simulink model "AirbrakeFlightSim"  (R2024b)
settings: Solver=ode45  StartTime=0.0  StopTime=18  FixedStep=0.001  RelTol=1e-4  AbsTol=1e-6
model workspace (MAT data in the model file):
  test = 1
undefined symbols (not defined in the file or in its folder): accelerometer, atm, dspblkCoreblockFVToolHelper, gcbh, gyroscope, model_g_mps2, true_g_mps2, wn, zeta
libraries: simulink x14, simulink_extras x10, matrix_library x2, slpidlib x1
(part 1 of 2)
settings Model: Creator=colin  LastModifiedBy=colin
settings SolverCC: AutoScaleAbsTol=off
settings DebuggingCC: UnderSpecifiedDimensionMsg=warning

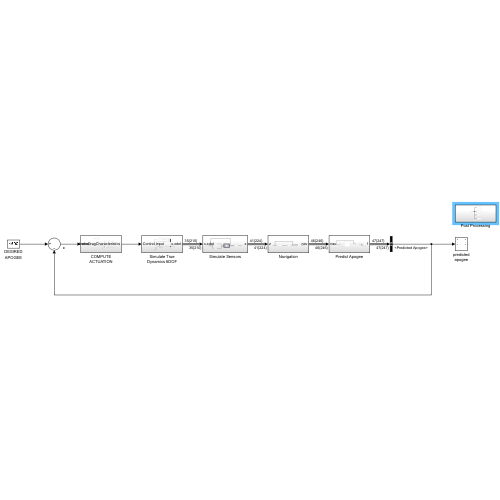
[thumbnail: Simulink's stored preview of the top-level diagram]
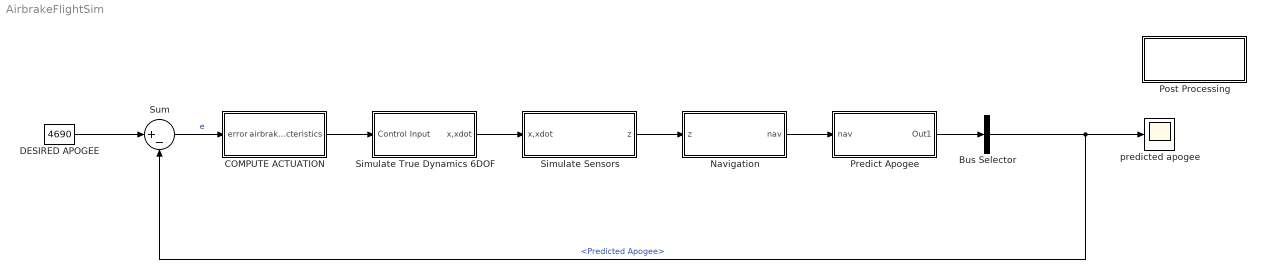
== system AirbrakeFlightSim ==
  Bus Selector : BusSelector  OutputSignals=Predicted Apogee
  COMPUTE ACTUATION : Subsystem
  DESIRED APOGEE : Constant  Value=4690
  Navigation : Subsystem
  Post Processing : Subsystem
  Predict Apogee : Subsystem
  Simulate Sensors : Subsystem
  Simulate True Dynamics 6DOF : Subsystem
  Sum : Sum  Inputs=|+-
  predicted apogee : Scope
  wires:
  DESIRED APOGEE/1 -> Sum/1
  Sum/1 -> COMPUTE ACTUATION/1(error)  "e"
  COMPUTE ACTUATION/1(airbrakeDragCharacteristics) -> Simulate True Dynamics 6DOF/1(Control Input)
  Simulate True Dynamics 6DOF/1(x,xdot) -> Simulate Sensors/1(x,xdot)
  Simulate Sensors/1(z) -> Navigation/1(z)
  Navigation/1(nav) -> Predict Apogee/1(nav)
  Bus Selector/1 -> predicted apogee/1, Sum/2  "<Predicted Apogee>"
  Predict Apogee/1(Out1) -> Bus Selector/1

== system AirbrakeFlightSim/COMPUTE ACTUATION ==
  error : Inport
  Add : Sum
  CONTROL SIGNAL : Scope
  CONTROLLER : slpidlib/PID Controller  Controller=PID  Form=Parallel  TimeDomain=Discrete-time  UseExternalTs=off  SampleTime=0.05  IntegratorMethod=Forward Euler  FilterMethod=Forward Euler  ControllerParametersSource=internal  P=10  I=1  UseKiTs=off  D=0  UseExternalDerivativeSource=off  N=0.01  UseFilter=on  TunerSelectOption=Frequency Response Based  InitialConditionSource=internal  InitialConditionForIntegrator=0  InitialConditionForFilter=0  DifferentiatorICPrevScaledInput=0  ExternalReset=none  TrackingMode=off  Kt=1  LimitOutput=off  SatLimitsSource=internal  UpperSaturationLimit=100  LowerSaturationLimit=0  LinearizeAsGain=on  AntiWindupMode=clamping  Kb=1  LimitIntegrator=off  UpperIntegratorSaturationLimit=inf  LowerIntegratorSaturationLimit=-inf  POutMin=[]  POutMax=[]  IOutMin=[]  IOutMax=[]  DOutMin=[]  DOutMax=[]  NOutMin=[]  NOutMax=[]  SumOutMin=[]  SumOutMax=[]  SaturationOutMin=[]  SaturationOutMax=[]  PParamMin=[]  PParamMax=[]  IParamMin=[]  IParamMax=[]  DParamMin=[]  DParamMax=[]  NParamMin=[]  NParamMax=[]  KbParamMin=[]  KbParamMax=[]  KtParamMin=[]  KtParamMax=[]  KbOutMin=[]  KbOutMax=[]  KtOutMin=[]  KtOutMax=[]  IntegratorOutMin=[]  IntegratorOutMax=[]  FilterOutMin=[]  FilterOutMax=[]  SumI1OutMin=[]  SumI1OutMax=[]  SumI2OutMin=[]  SumI2OutMax=[]  SumI3OutMin=[]  SumI3OutMax=[]  SumI4OutMin=[]  SumI4OutMax=[]  SumDOutMin=[]  SumDOutMax=[]  DifferentiatorOutMin=[]  DifferentiatorOutMax=[]  FilterDiffOutCoefMin=[]  FilterDiffOutCoefMax=[]  ReciprocalOutMin=[]  ReciprocalOutMax=[]  SumDenOutMin=[]  SumDenOutMax=[]  SumNumOutMin=[]  SumNumOutMax=[]  DivideOutMin=[]  DivideOutMax=[]  UdiffTsProdOutMin=[]  UdiffTsProdOutMax=[]  NTsProdOutMin=[]  NTsProdOutMax=[]  UintegralTsProdOutMin=[]  UintegralTsProdOutMax=[]  UngainTsProdOutMin=[]  UngainTsProdOutMax=[]  ClampingZeroOutDataTypeStr=Inherit: Inherit via back propagation  ClampingZeroOutMin=[]  ClampingZeroOutMax=[]  FilterDenConstantOutDataTypeStr=Inherit: Inherit via back propagation  FilterDenConstantOutMin=[]  FilterDenConstantOutMax=[]  PCopyOutDataTypeStr=Inherit: Inherit via back propagation  PCopyOutMin=[]  PCopyOutMax=[]  NCopyOutDataTypeStr=Inherit: Inherit via back propagation  NCopyOutMin=[]  NCopyOutMax=[]  IntegratorContinuousStateAttributes=''  IntegratorStateMustResolveToSignalObject=off  IntegratorRTWStateStorageClass=Auto  FilterContinuousStateAttributes=''  FilterStateMustResolveToSignalObject=off  FilterRTWStateStorageClass=Auto  ParallelPVariant=InternalParameters  IdealPVariant=Disabled  IVariant=InternalParameters  DVariant=InternalParameters  IntegratorVariant=Discrete  SatVariant=Disabled  AWVariant=Passthrough  PCopyVariant=Disabled  TRVariant=Disabled  FdbkBlocksVariant=Forward  IdealPFdbkVariant=Disabled  SatFdbkVariant=Disabled  DerivativeFilterVariant=ForwardEulerFilter  NVariant=InternalParameters  NCopyVariant=Disabled  FilterICVariant=InternalICsFilter  IntegratorICVariant=InternalICs  ExternalResetVariant=Disabled  TRSumVariant=Passthrough  SumFdbkVariant=Disabled  SumVariant=Sum_PID  TsampFilterVariant=InternalTs  TsampNgainVariant=Passthrough  TsampIntegralVariant=Disabled_SignalSpec  ExternalSaturationOutDataTypeStr=Inherit: Same as second input  DerivativeSourceVariant=ErrorSignal  PreIntVariant=InternalPreInt
  Cd*refArea2 : Constant  Value=0.00935787530743346
  DRAG : Scope
  ERROR SIGNAL : Scope
  GAIN-CONTROLLED SIGNAL : Scope
  Gain : Gain  Gain=-1
  Gain1 : Gain  Gain=-1e-4
  IDEAL DRAG : Scope
  Saturation1 : Saturate  UpperLimit=2*0.00935787530743346  LowerLimit=0.00935787530743346
  Switch1 : Switch  Criteria=u2 > Threshold  SaturateOnIntegerOverflow=off  InputSameDT=off
  airbrakeDragCharacteristics : Outport
  wires:
  CONTROLLER/1 -> Gain1/1, CONTROL SIGNAL/1
  Cd*refArea2/1 -> Add/2
  Gain1/1 -> GAIN-CONTROLLED SIGNAL/1, Add/1
  Add/1 -> Saturation1/1, IDEAL DRAG/1
  Saturation1/1 -> DRAG/1, airbrakeDragCharacteristics/1
  Gain/1 -> ERROR SIGNAL/1
  [motor_burnout] -> Switch1/2
  error/1 -> Switch1/1
  Switch1/1 -> CONTROLLER/1

== system AirbrakeFlightSim/Navigation ==
  z : Inport
  Compute Drag : Subsystem
  Dead Reckoning : Subsystem
  Reorganize : Subsystem
  nav : Outport
  wires:
  z/1 -> Dead Reckoning/1(z), Reorganize/1(z)
  Dead Reckoning/1(nav) -> Compute Drag/1(nav)
  Reorganize/1(Out1) -> nav/1
  Compute Drag/1(dragConstant) -> Reorganize/2(nav)

== system AirbrakeFlightSim/Post Processing ==
  Custom : Subsystem
  Navigation : Subsystem
  Navigation Error : Subsystem
  True Dynamics : Subsystem
  wires:
  [Master] -> True Dynamics/1(In1), Navigation/1(nav), Navigation Error/1(In1), Custom/1(In1)

== system AirbrakeFlightSim/Predict Apogee ==
  nav : Inport
  Bus Selector : BusSelector  OutputSignals=Navigation Data.Estimated Drag Constant,Navigation Data.NED.NED Velocity,Navigation Data.NED.NED Position
  PREDICT APOGEE : MATLAB Function  TreatAsAtomicUnit=on
  Reorganize : Subsystem
  Out1 : Outport
  tag scope: Master=global
  wires:
  Reorganize/1(Out1) -> Out1/1, [Master]
  PREDICT APOGEE/1(y) -> Reorganize/2(y)
  nav/1 -> Reorganize/1(nav), Bus Selector/1
  Bus Selector/3 -> PREDICT APOGEE/3(position)  "<NED Position>"
  Bus Selector/1 -> PREDICT APOGEE/1(dragConstant)  "<Estimated Drag Constant>"
  Bus Selector/2 -> PREDICT APOGEE/2(velocity)  "<NED Velocity>"

== system AirbrakeFlightSim/Simulate Sensors ==
  note: SELECT SENSOR MODE
  x,xdot : Inport
  Ideal Sensors : Subsystem
  Manual Switch : ManualSwitch
  Noisy Sensors : Subsystem
  Reorganize : Subsystem
  z : Outport
  wires:
  x,xdot/1 -> Noisy Sensors/1(x,xdot), Ideal Sensors/1(x,xdot), Reorganize/1(x,xdot)
  Ideal Sensors/1(meas) -> Manual Switch/2  "Ideal Measurements"
  Noisy Sensors/1(Measurements) -> Manual Switch/1
  Manual Switch/1 -> Reorganize/2(Measurements)  "Measurements"
  Reorganize/1(z) -> z/1

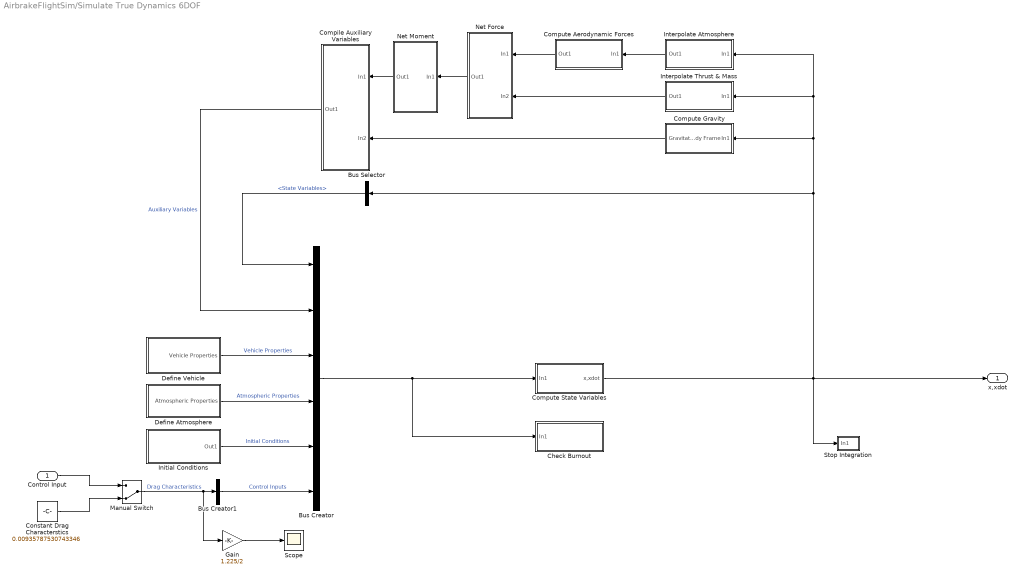
== system AirbrakeFlightSim/Simulate True Dynamics 6DOF ==
  Control Input : Inport
  Bus Creator : BusCreator  Inputs=State Variables,Auxiliary Variables,Vehicle Properties,Atmospheric Properties,Initial Conditions,Control Inputs
  Bus Creator1 : BusCreator  Inputs=Drag Characteristics
  Bus Selector : BusSelector  OutputSignals=State Variables
  Check Burnout : Subsystem
  Compile Auxiliary Variables : Subsystem
  Compute Aerodynamic Forces : Subsystem
  Compute Gravity : Subsystem
  Compute State Variables : Subsystem
  Constant Drag Characterstics : Constant  Value=0.00935787530743346
  Define Atmosphere : Subsystem
  Define Vehicle : Subsystem
  Gain : Gain  Gain=1.225/2
  Initial Conditions : Subsystem
  Interpolate Atmosphere : Subsystem
  Interpolate Thrust & Mass : Subsystem
  Manual Switch : ManualSwitch  CurrentSetting=0
  Net Force : Subsystem
  Net Moment : Subsystem
  Scope : Scope
  Stop Integration : Subsystem
  x,xdot : Outport
  wires:
  Compute Gravity/1(Gravitational Acceleration Vector in Body Frame) -> Compile Auxiliary Variables/2(In2)
  Define Vehicle/1(Vehicle Properties) -> Bus Creator/3  "Vehicle Properties"
  Initial Conditions/1(Out1) -> Bus Creator/5  "Initial Conditions"
  Bus Selector/1 -> Bus Creator/1  "<State Variables>"
  Compile Auxiliary Variables/1(Out1) -> Bus Creator/2  "Auxiliary Variables"
  Net Force/1(Out1) -> Net Moment/1(In1)
  Bus Creator/1 -> Compute State Variables/1(In1), Check Burnout/1(In1)
  Interpolate Thrust & Mass/1(Out1) -> Net Force/2(In2)
  Net Moment/1(Out1) -> Compile Auxiliary Variables/1(In1)
  Bus Creator1/1 -> Bus Creator/6  "Control Inputs"
  Manual Switch/1 -> Gain/1, Bus Creator1/1  "Drag Characteristics"
  Compute Aerodynamic Forces/1(Out1) -> Net Force/1(In1)
  Define Atmosphere/1(Atmospheric Properties) -> Bus Creator/4  "Atmospheric Properties"
  Interpolate Atmosphere/1(Out1) -> Compute Aerodynamic Forces/1(In1)
  Control Input/1 -> Manual Switch/1
  Constant Drag Characterstics/1 -> Manual Switch/2
  Compute State Variables/1(x,xdot) -> x,xdot/1, Stop Integration/1(In1), Bus Selector/1, Compute Gravity/1(In1), Interpolate Thrust & Mass/1(In1), Interpolate Atmosphere/1(In1)
  Gain/1 -> Scope/1

== system AirbrakeFlightSim/Navigation/Compute Drag ==
  nav : Inport
  Bus Selector : BusSelector  OutputSignals=NED.NED Acceleration,NED.NED Velocity
  MATLAB Function : MATLAB Function  TreatAsAtomicUnit=on
  Reorganize : Subsystem
  g NED1 : Constant  Value=[0 0 9.81]'
  dragConstant : Outport
  wires:
  nav/1 -> Bus Selector/1, Reorganize/1(nav)
  Reorganize/1(dragConstant) -> dragConstant/1
  MATLAB Function/1(drag_const) -> Reorganize/2(y)
  Bus Selector/1 -> MATLAB Function/1(a_ned_mps2)  "<NED Acceleration>"
  Bus Selector/2 -> MATLAB Function/2(v_ned_mps)  "<NED Velocity>"
  g NED1/1 -> MATLAB Function/3(gvec_ned)

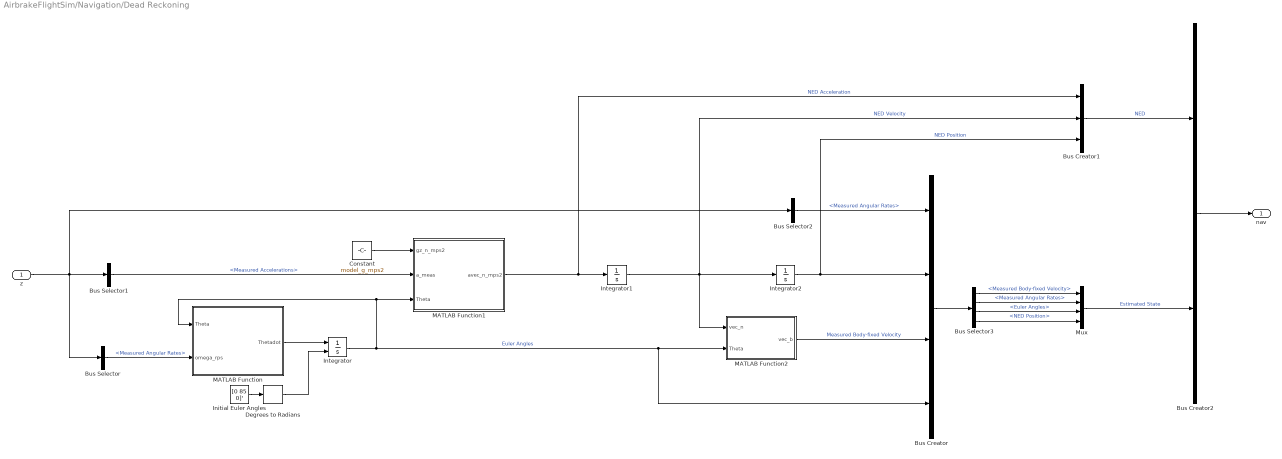
== system AirbrakeFlightSim/Navigation/Dead Reckoning ==
  z : Inport
  Bus Creator : BusCreator  Inputs=4
  Bus Creator1 : BusCreator  Inputs=3
  Bus Creator2 : BusCreator  Inputs=2
  Bus Selector : BusSelector  OutputSignals=Measurements.Measured Angular Rates
  Bus Selector1 : BusSelector  OutputSignals=Measurements.Measured Accelerations
  Bus Selector2 : BusSelector  OutputSignals=Measurements.Measured Angular Rates
  Bus Selector3 : BusSelector  OutputSignals=Measured Body-fixed Velocity,Measured Angular Rates,Euler Angles,NED Position
  Constant : Constant  Value=model_g_mps2
  Degrees to Radians : simulink_extras/Transformations/Degrees to Radians
  Initial Euler Angles : Constant  Value=[0 85 0]'
  Integrator : Integrator  InitialConditionSource=external
  Integrator1 : Integrator
  Integrator2 : Integrator
  MATLAB Function : MATLAB Function  TreatAsAtomicUnit=on
  MATLAB Function1 : MATLAB Function  TreatAsAtomicUnit=on
  MATLAB Function2 : MATLAB Function  TreatAsAtomicUnit=on
  Mux : Mux
  nav : Outport
  wires:
  Integrator2/1 -> Bus Creator/2, Bus Creator1/3  "NED Position"
  Integrator1/1 -> Bus Creator1/2, MATLAB Function2/1(vec_n), Integrator2/1  "NED Velocity"
  Integrator/1 -> Bus Creator/4, MATLAB Function2/2(Theta), MATLAB Function/1(Theta), MATLAB Function1/3(Theta)  "Euler Angles"
  Bus Selector3/4 -> Mux/4  "<NED Position>"
  MATLAB Function1/1(avec_n_mps2) -> Integrator1/1, Bus Creator1/1  "NED Acceleration"
  Degrees to Radians/1 -> Integrator/2
  z/1 -> Bus Selector2/1, Bus Selector1/1, Bus Selector/1
  Bus Creator/1 -> Bus Selector3/1
  Initial Euler Angles/1 -> Degrees to Radians/1
  Bus Selector2/1 -> Bus Creator/1  "<Measured Angular Rates>"
  MATLAB Function/1(Thetadot) -> Integrator/1
  Bus Selector/1 -> MATLAB Function/2(omega_rps)  "<Measured Angular Rates>"
  Bus Selector1/1 -> MATLAB Function1/2(a_meas)  "<Measured Accelerations>"
  Bus Selector3/3 -> Mux/3  "<Euler Angles>"
  MATLAB Function2/1(vec_b) -> Bus Creator/3  "Measured Body-fixed Velocity"
  Bus Selector3/2 -> Mux/2  "<Measured Angular Rates>"
  Bus Selector3/1 -> Mux/1  "<Measured Body-fixed Velocity>"
  Bus Creator1/1 -> Bus Creator2/1  "NED"
  Mux/1 -> Bus Creator2/2  "Estimated State"
  Bus Creator2/1 -> nav/1
  Constant/1 -> MATLAB Function1/1(gz_n_mps2)

== system AirbrakeFlightSim/Navigation/Reorganize ==
  z : Inport
  nav : Inport  Port=2
  Bus Creator : BusCreator  Inputs=8
  Bus Selector : BusSelector  OutputSignals=State Variables,State Derivatives,Vehicle Properties,Atmospheric Properties,Control Inputs,Auxiliary Variables,Measurements
  Out1 : Outport
  wires:
  z/1 -> Bus Selector/1
  Bus Selector/1 -> Bus Creator/1  "<State Variables>"
  Bus Selector/2 -> Bus Creator/2  "<State Derivatives>"
  Bus Selector/3 -> Bus Creator/3  "<Vehicle Properties>"
  Bus Selector/4 -> Bus Creator/4  "<Atmospheric Properties>"
  Bus Selector/5 -> Bus Creator/5  "<Control Inputs>"
  Bus Selector/6 -> Bus Creator/6  "<Auxiliary Variables>"
  Bus Selector/7 -> Bus Creator/7  "<Measurements>"
  nav/1 -> Bus Creator/8  "Navigation Data"
  Bus Creator/1 -> Out1/1

== system AirbrakeFlightSim/Post Processing/Custom ==
  In1 : Inport
  Bus Selector : BusSelector  OutputSignals=State Variables,State Derivatives,Auxiliary Variables.Simulation Time,Measurements.Measured GPS Position,Measurements.Measured GPS Velocity,Measurements.Measured Heading,Measurements.Measured Altitude,Measurements.Measured Angular Rates,Measurements.Measured Accelerations
  To Workspace : ToWorkspace  VariableName=x  SaveFormat=Timeseries  SampleTime=-1
  To Workspace1 : ToWorkspace  VariableName=xdot  SaveFormat=Timeseries  SampleTime=-1
  To Workspace2 : ToWorkspace  VariableName=t  SaveFormat=Timeseries  SampleTime=-1
  To Workspace3 : ToWorkspace  VariableName=gps_pos  SaveFormat=Timeseries  SampleTime=-1
  To Workspace4 : ToWorkspace  VariableName=gps_vel  SaveFormat=Timeseries  SampleTime=-1
  To Workspace5 : ToWorkspace  VariableName=mag_yaw  SaveFormat=Timeseries  SampleTime=-1
  To Workspace6 : ToWorkspace  VariableName=alti_pd  SaveFormat=Timeseries  SampleTime=-1
  To Workspace7 : ToWorkspace  VariableName=imu_pqr  SaveFormat=Timeseries  SampleTime=-1
  To Workspace8 : ToWorkspace  VariableName=imu_accel  SaveFormat=Timeseries  SampleTime=-1
  wires:
  In1/1 -> Bus Selector/1
  Bus Selector/1 -> To Workspace/1  "<State Variables>"
  Bus Selector/2 -> To Workspace1/1  "<State Derivatives>"
  Bus Selector/3 -> To Workspace2/1  "<Simulation Time>"
  Bus Selector/4 -> To Workspace3/1  "<Measured GPS Position>"
  Bus Selector/5 -> To Workspace4/1  "<Measured GPS Velocity>"
  Bus Selector/6 -> To Workspace5/1  "<Measured Heading>"
  Bus Selector/7 -> To Workspace6/1  "<Measured Altitude>"
  Bus Selector/8 -> To Workspace7/1  "<Measured Angular Rates>"
  Bus Selector/9 -> To Workspace8/1  "<Measured Accelerations>"

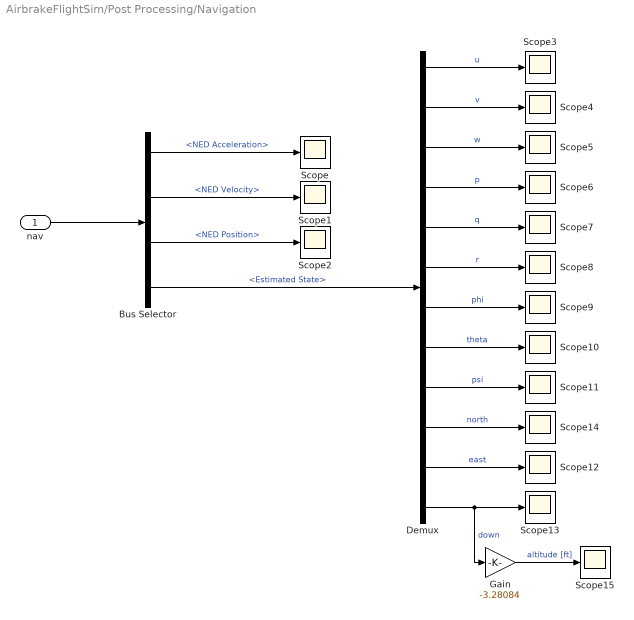
== system AirbrakeFlightSim/Post Processing/Navigation ==
  nav : Inport
  Bus Selector : BusSelector  OutputSignals=Navigation Data.NED.NED Acceleration,Navigation Data.NED.NED Velocity,Navigation Data.NED.NED Position,Navigation Data.Estimated State
  Demux : Demux  Outputs=12
  Gain : Gain  Gain=-3.28084
  Scope{,1..15} (16 alike) : Scope
  wires:
  Demux/8 -> Scope10/1  "theta"
  Demux/6 -> Scope8/1  "r"
  Demux/4 -> Scope6/1  "p"
  Demux/11 -> Scope12/1  "east"
  nav/1 -> Bus Selector/1
  Demux/5 -> Scope7/1  "q"
  Demux/3 -> Scope5/1  "w"
  Demux/2 -> Scope4/1  "v"
  Demux/10 -> Scope14/1  "north"
  Bus Selector/2 -> Scope1/1  "<NED Velocity>"
  Demux/7 -> Scope9/1  "phi"
  Demux/12 -> Gain/1, Scope13/1  "down"
  Demux/1 -> Scope3/1  "u"
  Bus Selector/4 -> Demux/1  "<Estimated State>"
  Bus Selector/1 -> Scope/1  "<NED Acceleration>"
  Demux/9 -> Scope11/1  "psi"
  Bus Selector/3 -> Scope2/1  "<NED Position>"
  Gain/1 -> Scope15/1  "altitude [ft]"

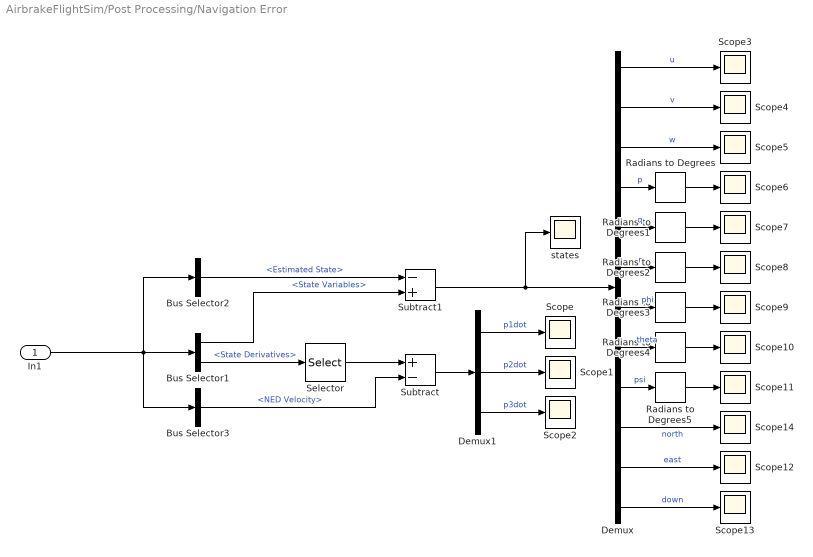
== system AirbrakeFlightSim/Post Processing/Navigation Error ==
  In1 : Inport
  Bus Selector1 : BusSelector  OutputSignals=State Variables,State Derivatives
  Bus Selector2 : BusSelector  OutputSignals=Navigation Data.Estimated State
  Bus Selector3 : BusSelector  OutputSignals=Navigation Data.NED.NED Velocity
  Demux : Demux  Outputs=12
  Demux1 : Demux  Outputs=3
  Radians to Degrees{,1..5} (6 alike) : simulink_extras/Transformations/Radians to Degrees
  Scope{,1..14} (15 alike) : Scope
  Selector : Selector  InputPortWidth=12  IndexOptions=Index vector (dialog)  Indices=[10 11 12]  OutputSizes=1
  Subtract : Sum  Inputs=+-
  Subtract1 : Sum  Inputs=-+
  states : Scope
  wires:
  In1/1 -> Bus Selector3/1, Bus Selector2/1, Bus Selector1/1
  Demux/4 -> Radians to Degrees/1  "p"
  Demux/12 -> Scope13/1  "down"
  Bus Selector1/2 -> Selector/1  "<State Derivatives>"
  Bus Selector2/1 -> Subtract1/1  "<Estimated State>"
  Subtract/1 -> Demux1/1
  Demux/5 -> Radians to Degrees1/1  "q"
  Demux/9 -> Radians to Degrees5/1  "psi"
  Bus Selector3/1 -> Subtract/2  "<NED Velocity>"
  Demux/3 -> Scope5/1  "w"
  Demux/1 -> Scope3/1  "u"
  Demux1/2 -> Scope1/1  "p2dot"
  Demux1/1 -> Scope/1  "p1dot"
  Demux1/3 -> Scope2/1  "p3dot"
  Demux/2 -> Scope4/1  "v"
  Demux/10 -> Scope14/1  "north"
  Subtract1/1 -> states/1, Demux/1
  Demux/6 -> Radians to Degrees2/1  "r"
  Bus Selector1/1 -> Subtract1/2  "<State Variables>"
  Demux/11 -> Scope12/1  "east"
  Selector/1 -> Subtract/1
  Demux/7 -> Radians to Degrees3/1  "phi"
  Demux/8 -> Radians to Degrees4/1  "theta"
  Radians to Degrees/1 -> Scope6/1
  Radians to Degrees1/1 -> Scope7/1
  Radians to Degrees2/1 -> Scope8/1
  Radians to Degrees3/1 -> Scope9/1
  Radians to Degrees4/1 -> Scope10/1
  Radians to Degrees5/1 -> Scope11/1

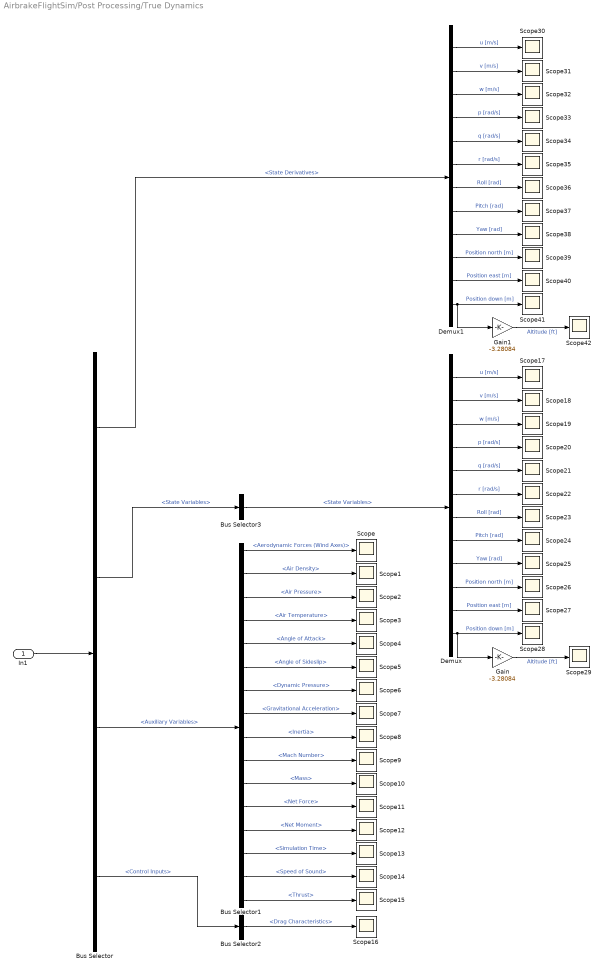
== system AirbrakeFlightSim/Post Processing/True Dynamics ==
  In1 : Inport
  Bus Selector : BusSelector  OutputSignals=State Derivatives,State Variables,Auxiliary Variables,Control Inputs
  Bus Selector1 : BusSelector  OutputSignals=Aerodynamic Forces (Wind Axes),Air Density,Air Pressure,Air Temperature,Angle of Attack,Angle of Sideslip,Dynamic Pressure,Gravitational Acceleration,Inertia,Mach Number,Mass,Net Force,Net Moment,Simulation Time,Speed of Sound,Thrust
  Bus Selector2 : BusSelector  OutputSignals=Drag Characteristics
  Bus Selector3 : BusSelector  OutputSignals=State Variables
  Demux : Demux  Outputs=12
  Demux1 : Demux  Outputs=12
  Gain : Gain  Gain=-3.28084
  Gain1 : Gain  Gain=-3.28084
  Scope{,1..42} (43 alike) : Scope
  wires:
  In1/1 -> Bus Selector/1
  Bus Selector/3 -> Bus Selector1/1  "<Auxiliary Variables>"
  Bus Selector/4 -> Bus Selector2/1  "<Control Inputs>"
  Bus Selector/2 -> Bus Selector3/1  "<State Variables>"
  Bus Selector1/1 -> Scope/1  "<Aerodynamic Forces (Wind Axes)>"
  Bus Selector1/2 -> Scope1/1  "<Air Density>"
  Bus Selector1/3 -> Scope2/1  "<Air Pressure>"
  Bus Selector3/1 -> Demux/1  "<State Variables>"
  Bus Selector2/1 -> Scope16/1  "<Drag Characteristics>"
  Bus Selector1/16 -> Scope15/1  "<Thrust>"
  Bus Selector1/15 -> Scope14/1  "<Speed of Sound>"
  Bus Selector1/14 -> Scope13/1  "<Simulation Time>"
  Bus Selector1/13 -> Scope12/1  "<Net Moment>"
  Bus Selector1/12 -> Scope11/1  "<Net Force>"
  Bus Selector1/11 -> Scope10/1  "<Mass>"
  Bus Selector1/10 -> Scope9/1  "<Mach Number>"
  Bus Selector1/9 -> Scope8/1  "<Inertia>"
  Bus Selector1/7 -> Scope6/1  "<Dynamic Pressure>"
  Bus Selector1/6 -> Scope5/1  "<Angle of Sideslip>"
  Bus Selector1/5 -> Scope4/1  "<Angle of Attack>"
  Bus Selector1/4 -> Scope3/1  "<Air Temperature>"
  Demux/1 -> Scope17/1  "u [m/s]"
  Demux/2 -> Scope18/1  "v [m/s]"
  Demux/3 -> Scope19/1  "w [m/s]"
  Demux/4 -> Scope20/1  "p [rad/s]"
  Demux/5 -> Scope21/1  "q [rad/s]"
  Demux/6 -> Scope22/1  "r [rad/s]"
  Demux/7 -> Scope23/1  "Roll [rad]"
  Demux/8 -> Scope24/1  "Pitch [rad]"
  Demux/9 -> Scope25/1  "Yaw [rad]"
  Demux/10 -> Scope26/1  "Position north [m]"
  Demux/11 -> Scope27/1  "Position east [m]"
  Demux/12 -> Scope28/1, Gain/1  "Position down [m]"
  Gain/1 -> Scope29/1  "Altitude [ft]"
  Bus Selector1/8 -> Scope7/1  "<Gravitational Acceleration>"
  Demux1/11 -> Scope40/1  "Position east [m]"
  Demux1/12 -> Scope41/1, Gain1/1  "Position down [m]"
  Demux1/2 -> Scope31/1  "v [m/s]"
  Demux1/9 -> Scope38/1  "Yaw [rad]"
  Demux1/7 -> Scope36/1  "Roll [rad]"
  Demux1/10 -> Scope39/1  "Position north [m]"
  Demux1/3 -> Scope32/1  "w [m/s]"
  Demux1/6 -> Scope35/1  "r [rad/s]"
  Demux1/5 -> Scope34/1  "q [rad/s]"
  Demux1/1 -> Scope30/1  "u [m/s]"
  Gain1/1 -> Scope42/1  "Altitude [ft]"
  Demux1/4 -> Scope33/1  "p [rad/s]"
  Demux1/8 -> Scope37/1  "Pitch [rad]"
  Bus Selector/1 -> Demux1/1  "<State Derivatives>"

== system AirbrakeFlightSim/Predict Apogee/Reorganize ==
  nav : Inport
  y : Inport  Port=2
  Bus Creator : BusCreator  Inputs=9
  Bus Selector : BusSelector  OutputSignals=State Variables,State Derivatives,Vehicle Properties,Atmospheric Properties,Control Inputs,Auxiliary Variables,Measurements,Navigation Data
  Out1 : Outport
  wires:
  nav/1 -> Bus Selector/1
  Bus Selector/1 -> Bus Creator/1  "<State Variables>"
  Bus Selector/2 -> Bus Creator/2  "<State Derivatives>"
  Bus Selector/3 -> Bus Creator/3  "<Vehicle Properties>"
  Bus Selector/4 -> Bus Creator/4  "<Atmospheric Properties>"
  Bus Selector/5 -> Bus Creator/5  "<Control Inputs>"
  Bus Selector/6 -> Bus Creator/6  "<Auxiliary Variables>"
  Bus Selector/8 -> Bus Creator/8  "<Navigation Data>"
  Bus Selector/7 -> Bus Creator/7  "<Measurements>"
  y/1 -> Bus Creator/9  "Predicted Apogee"
  Bus Creator/1 -> Out1/1

== system AirbrakeFlightSim/Simulate Sensors/Ideal Sensors ==
  x,xdot : Inport
  Altimeter : Subsystem
  Bus Creator : BusCreator  Inputs=6
  Bus Selector : BusSelector  OutputSignals=State Variables,State Derivatives
  CG to Accelerometer Position Vector [m] : Constant  Value=[0.2 0.05 -0.05]
  Constant : Constant  Value=true_g_mps2
  GPS : Subsystem
  MATLAB Function : MATLAB Function  TreatAsAtomicUnit=on
  Magnetometer : Subsystem
  Selector1 : Selector  InputPortWidth=12  IndexOptions=Index vector (dialog)  Indices=[4 5 6]  OutputSizes=1
  meas : Outport
  wires:
  x,xdot/1 -> GPS/1(x,xdot), Magnetometer/1(x,xdot), Altimeter/1(x,xdot), Bus Selector/1
  Bus Selector/1 -> Selector1/1, MATLAB Function/1(x)  "<State Variables>"
  Bus Selector/2 -> MATLAB Function/2(xdot)  "<State Derivatives>"
  CG to Accelerometer Position Vector [m]/1 -> MATLAB Function/3(r_b_sensor)
  Selector1/1 -> Bus Creator/5  "Measured Angular Rates"
  MATLAB Function/1(astar) -> Bus Creator/6  "Measured Accelerations"
  Bus Creator/1 -> meas/1
  Constant/1 -> MATLAB Function/4(gz_n_mps2)
  Altimeter/1(altitudehat) -> Bus Creator/4  "Measured Altitude"
  Magnetometer/1(headinghat) -> Bus Creator/3  "Measured Heading"
  GPS/2(vhat) -> Bus Creator/2  "Measured GPS Velocity"
  GPS/1(rhat) -> Bus Creator/1  "Measured GPS Position"

== system AirbrakeFlightSim/Simulate Sensors/Noisy Sensors ==
  note: Need to adjust these to be asynchronous
  x,xdot : Inport
  Accelerometer : Subsystem
  Altimeter : Subsystem
  Bus Creator : BusCreator  Inputs=6
  GPS : Subsystem
  Gyroscope : Subsystem
  Magnetometer : Subsystem
  Measurements : Outport
  wires:
  Altimeter/1(altitudehat) -> Bus Creator/4  "Measured Altitude"
  Gyroscope/1(omegahat) -> Bus Creator/5  "Measured Angular Rates"
  Accelerometer/1(ahat) -> Bus Creator/6  "Measured Accelerations"
  x,xdot/1 -> Accelerometer/1(x,xdot), Gyroscope/1(x,xdot), GPS/1(x,xdot), Magnetometer/1(x,xdot), Altimeter/1(x,xdot)
  Bus Creator/1 -> Measurements/1  "Measurements"
  Magnetometer/1(headinghat) -> Bus Creator/3  "Measured Heading"
  GPS/1(rhat) -> Bus Creator/1  "Measured GPS Position"
  GPS/2(vhat) -> Bus Creator/2  "Measured GPS Velocity"

== system AirbrakeFlightSim/Simulate Sensors/Reorganize ==
  x,xdot : Inport
  Measurements : Inport  Port=2
  Bus Creator : BusCreator  Inputs=7
  Bus Selector : BusSelector  OutputSignals=State Variables,State Derivatives,Vehicle Properties,Atmospheric Properties,Control Inputs,Auxiliary Variables
  z : Outport
  wires:
  x,xdot/1 -> Bus Selector/1
  Bus Selector/1 -> Bus Creator/1  "<State Variables>"
  Bus Selector/2 -> Bus Creator/2  "<State Derivatives>"
  Bus Selector/3 -> Bus Creator/3  "<Vehicle Properties>"
  Bus Selector/4 -> Bus Creator/4  "<Atmospheric Properties>"
  Bus Selector/5 -> Bus Creator/5  "<Control Inputs>"
  Bus Selector/6 -> Bus Creator/6  "<Auxiliary Variables>"
  Measurements/1 -> Bus Creator/7
  Bus Creator/1 -> z/1

== system AirbrakeFlightSim/Simulate True Dynamics 6DOF/Check Burnout ==
  In1 : Inport
  Add : Sum
  Add Constant : Bias  Bias=-0.1  SaturateOnIntegerOverflow=off
  Bus Selector : BusSelector  OutputSignals=Vehicle Properties.Motor Time Breakpoints,Auxiliary Variables.Simulation Time
  Gain : Gain  Gain=-1
  Selector : Selector  InputPortWidth=20  IndexOptions=Index vector (dialog)  Indices=[20]  OutputSizes=1
  tag scope: motor_burnout=global
  wires:
  Selector/1 -> Add/1
  Add/1 -> Add Constant/1  "Time Since Burnout"
  Bus Selector/1 -> Gain/1  "<Motor Time Breakpoints>"
  In1/1 -> Bus Selector/1
  Gain/1 -> Selector/1
  Bus Selector/2 -> Add/2  "<Simulation Time>"
  Add Constant/1 -> [motor_burnout]

== system AirbrakeFlightSim/Simulate True Dynamics 6DOF/Compile Auxiliary Variables ==
  In1 : Inport
  In2 : Inport  Port=2
  Bus Creator : BusCreator  Inputs=16
  Bus Selector : BusSelector  OutputSignals=Aerodynamic Forces (Wind Axes),Air Density,Air Pressure,Air Temperature,Angle of Attack,Angle of Sideslip,Dynamic Pressure,Inertia,Mach Number,Mass,Net Force,Net Moment,Simulation Time,Speed of Sound,Thrust
  Out1 : Outport
  wires:
  In1/1 -> Bus Selector/1
  In2/1 -> Bus Creator/8  "Gravitational Acceleration"
  Bus Selector/15 -> Bus Creator/16  "<Thrust>"
  Bus Selector/1 -> Bus Creator/1  "<Aerodynamic Forces (Wind Axes)>"
  Bus Selector/2 -> Bus Creator/2  "<Air Density>"
  Bus Selector/3 -> Bus Creator/3  "<Air Pressure>"
  Bus Selector/4 -> Bus Creator/4  "<Air Temperature>"
  Bus Selector/5 -> Bus Creator/5  "<Angle of Attack>"
  Bus Selector/6 -> Bus Creator/6  "<Angle of Sideslip>"
  Bus Selector/7 -> Bus Creator/7  "<Dynamic Pressure>"
  Bus Selector/8 -> Bus Creator/9  "<Inertia>"
  Bus Selector/9 -> Bus Creator/10  "<Mach Number>"
  Bus Selector/10 -> Bus Creator/11  "<Mass>"
  Bus Selector/11 -> Bus Creator/12  "<Net Force>"
  Bus Selector/12 -> Bus Creator/13  "<Net Moment>"
  Bus Selector/13 -> Bus Creator/14  "<Simulation Time>"
  Bus Selector/14 -> Bus Creator/15  "<Speed of Sound>"
  Bus Creator/1 -> Out1/1

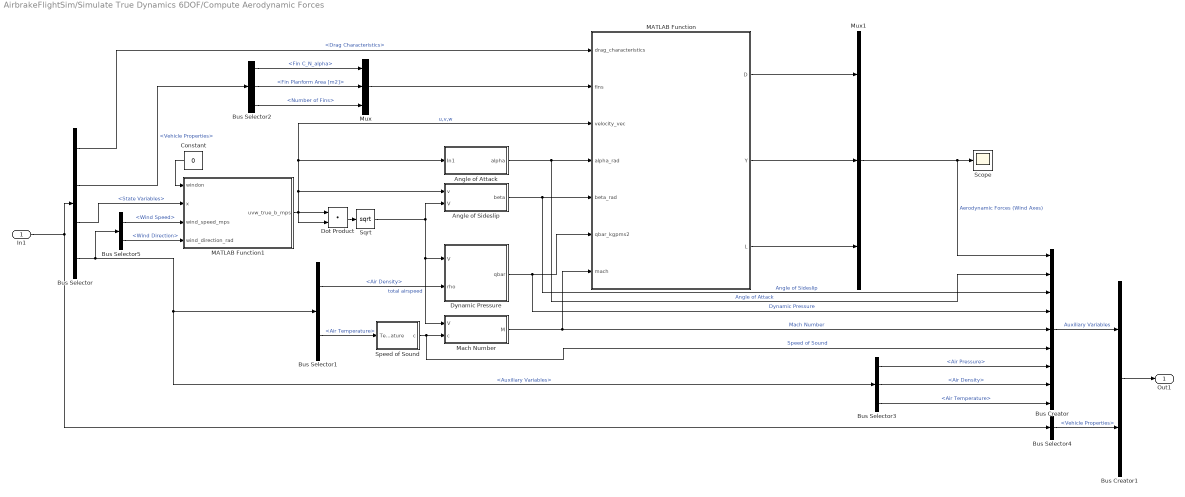
== system AirbrakeFlightSim/Simulate True Dynamics 6DOF/Compute Aerodynamic Forces ==
  In1 : Inport
  Angle of Attack : Subsystem
  Angle of Sideslip : Subsystem
  Bus Creator : BusCreator  Inputs=Aerodynamic Forces (Wind Axes),Angle of Attack,Angle of Sideslip,Dynamic Pressure,Mach Number,Speed of Sound,Air Pressure,Air Density,Air Temperature
  Bus Creator1 : BusCreator  Inputs=Auxiliary Variables,Vehicle Properties
  Bus Selector : BusSelector  OutputSignals=Control Inputs.Drag Characteristics,Vehicle Properties,State Variables,Auxiliary Variables
  Bus Selector1 : BusSelector  OutputSignals=Air Density,Air Temperature
  Bus Selector2 : BusSelector  OutputSignals=Fin C_N_alpha,Fin Planform Area [m2],Number of Fins
  Bus Selector3 : BusSelector  OutputSignals=Air Pressure,Air Density,Air Temperature
  Bus Selector4 : BusSelector  OutputSignals=Vehicle Properties
  Bus Selector5 : BusSelector  OutputSignals=Wind Speed,Wind Direction
  Constant : Constant  Value=0
  Dot Product : DotProduct  OutDataTypeStr=Inherit: Inherit via internal rule
  Dynamic Pressure : Subsystem
  MATLAB Function : MATLAB Function  TreatAsAtomicUnit=on
  MATLAB Function1 : MATLAB Function  TreatAsAtomicUnit=on
  Mach Number : Subsystem
  Mux : Mux  Inputs=3
  Mux1 : Mux  Inputs=3
  Scope : Scope
  Speed of Sound : Subsystem
  Sqrt : Sqrt
  Out1 : Outport
  wires:
  In1/1 -> Bus Selector4/1, Bus Selector/1
  MATLAB Function1/1(uvw_true_b_mps) -> Dot Product/2, MATLAB Function/3(velocity_vec), Angle of Attack/1(In1), Angle of Sideslip/1(v), Dot Product/1  "u,v,w"
  Sqrt/1 -> Dynamic Pressure/1(V), Mach Number/1(V), Angle of Sideslip/2(V)  "total airspeed"
  Dot Product/1 -> Sqrt/1
  Speed of Sound/1(c) -> Mach Number/2(c), Bus Creator/6  "Speed of Sound"
  Bus Selector/4 -> Bus Selector1/1, Bus Selector3/1, Bus Selector5/1  "<Auxiliary Variables>"
  Bus Selector1/1 -> Dynamic Pressure/2(rho)  "<Air Density>"
  Bus Selector1/2 -> Speed of Sound/1(Temperature)  "<Air Temperature>"
  Bus Selector/2 -> Bus Selector2/1  "<Vehicle Properties>"
  Angle of Attack/1(alpha) -> Bus Creator/2, MATLAB Function/4(alpha_rad)  "Angle of Attack"
  Angle of Sideslip/1(beta) -> Bus Creator/3, MATLAB Function/5(beta_rad)  "Angle of Sideslip"
  Dynamic Pressure/1(qbar) -> Bus Creator/4, MATLAB Function/6(qbar_kgpms2)  "Dynamic Pressure"
  Mach Number/1(M) -> Bus Creator/5, MATLAB Function/7(mach)  "Mach Number"
  Bus Selector2/3 -> Mux/3  "<Number of Fins>"
  Bus Selector2/2 -> Mux/2  "<Fin Planform Area [m2]>"
  Bus Selector2/1 -> Mux/1  "<Fin C_N_alpha>"
  Mux/1 -> MATLAB Function/2(fins)
  Bus Selector/1 -> MATLAB Function/1(drag_characteristics)  "<Drag Characteristics>"
  MATLAB Function/3(L) -> Mux1/3
  MATLAB Function/2(Y) -> Mux1/2
  MATLAB Function/1(D) -> Mux1/1
  Mux1/1 -> Scope/1, Bus Creator/1  "Aerodynamic Forces (Wind Axes)"
  Bus Selector3/1 -> Bus Creator/7  "<Air Pressure>"
  Bus Selector3/2 -> Bus Creator/8  "<Air Density>"
  Bus Selector3/3 -> Bus Creator/9  "<Air Temperature>"
  Bus Selector4/1 -> Bus Creator1/2  "<Vehicle Properties>"
  Bus Creator/1 -> Bus Creator1/1  "Auxiliary Variables"
  Bus Creator1/1 -> Out1/1
  Bus Selector/3 -> MATLAB Function1/2(x)  "<State Variables>"
  Bus Selector5/2 -> MATLAB Function1/4(wind_direction_rad)  "<Wind Direction>"
  Bus Selector5/1 -> MATLAB Function1/3(wind_speed_mps)  "<Wind Speed>"
  Constant/1 -> MATLAB Function1/1(windon)

== system AirbrakeFlightSim/Simulate True Dynamics 6DOF/Compute Gravity ==
  note: DCM_n2b_13
  note: NED to Body-Fixed
  note: Theta (Pitch) [rad]
  note: Phi (Roll) [rad]
  note: DCM_n2b_23
  note: DCM_n2b_33
  In1 : Inport
  Bus Selector : BusSelector  OutputSignals=State Variables
  Cos : Trigonometry  Operator=cos
  Cos1 : Trigonometry  Operator=cos
  Demux : Demux  Outputs=12
  Gain : Gain  Gain=-1
  Gain1 : Gain  Gain=true_g_mps2
  Gain2 : Gain  Gain=true_g_mps2
  Gain3 : Gain  Gain=true_g_mps2
  Mux : Mux  Inputs=3
  Product : Product
  Product1 : Product
  Sin : Trigonometry
  Sin1 : Trigonometry
  Gravitational Acceleration Vector in Body Frame : Outport
  wires:
  In1/1 -> Bus Selector/1
  Bus Selector/1 -> Demux/1  "<State Variables>"
  Demux/8 -> Cos1/1, Sin1/1
  Demux/7 -> Sin/1, Cos/1
  Sin1/1 -> Gain/1
  Sin/1 -> Product/1
  Cos1/1 -> Product1/1, Product/2
  Cos/1 -> Product1/2
  Gain/1 -> Gain1/1
  Product/1 -> Gain2/1
  Product1/1 -> Gain3/1
  Gain1/1 -> Mux/1
  Gain2/1 -> Mux/2
  Gain3/1 -> Mux/3
  Mux/1 -> Gravitational Acceleration Vector in Body Frame/1

== system AirbrakeFlightSim/Simulate True Dynamics 6DOF/Compute State Variables ==
  In1 : Inport
  Bus Creator1 : BusCreator  Inputs=6
  Bus Selector : BusSelector  OutputSignals=Vehicle Properties,Atmospheric Properties,Control Inputs,Auxiliary Variables
  Bus Selector1 : BusSelector  OutputSignals=State Variables,Auxiliary Variables.Net Force,Auxiliary Variables.Net Moment,Auxiliary Variables.Inertia,Auxiliary Variables.Mass,Auxiliary Variables.Gravitational Acceleration
  Bus Selector2 : BusSelector  OutputSignals=Initial Conditions.Initial State
  Integrator : Integrator  InitialConditionSource=external
  MATLAB Function : MATLAB Function  TreatAsAtomicUnit=on
  x,xdot : Outport
  wires:
  In1/1 -> Bus Selector/1, Bus Selector2/1, Bus Selector1/1
  Bus Creator1/1 -> x,xdot/1
  Bus Selector/1 -> Bus Creator1/3  "<Vehicle Properties>"
  Bus Selector/2 -> Bus Creator1/4  "<Atmospheric Properties>"
  Bus Selector/3 -> Bus Creator1/5  "<Control Inputs>"
  Bus Selector1/6 -> MATLAB Function/6(gvec_b_mps2)  "<Gravitational Acceleration>"
  Bus Selector1/5 -> MATLAB Function/5(m_kg)  "<Mass>"
  Bus Selector1/4 -> MATLAB Function/4(J_tensor_b_kgm2)  "<Inertia>"
  Bus Selector1/3 -> MATLAB Function/3(Mvec_b_N)  "<Net Moment>"
  Bus Selector1/2 -> MATLAB Function/2(Fvec_b_N)  "<Net Force>"
  Bus Selector1/1 -> MATLAB Function/1(x)  "<State Variables>"
  MATLAB Function/1(xdot) -> Integrator/1, Bus Creator1/2  "State Derivatives"
  Integrator/1 -> Bus Creator1/1  "State Variables"
  Bus Selector2/1 -> Integrator/2  "<Initial State>"
  Bus Selector/4 -> Bus Creator1/6  "<Auxiliary Variables>"

== system AirbrakeFlightSim/Simulate True Dynamics 6DOF/Define Atmosphere ==
  Bus Creator : BusCreator  Inputs=6
  Constant : Constant  Value=atm.elevation
  Constant1 : Constant  Value=atm.heights
  Constant2 : Constant  Value=atm.pressures
  Constant3 : Constant  Value=atm.temperatures
  Constant4 : Constant  Value=atm.wind_directions
  Constant5 : Constant  Value=atm.wind_speeds
  Atmospheric Properties : Outport
  wires:
  Bus Creator/1 -> Atmospheric Properties/1
  Constant/1 -> Bus Creator/1  "Local Elevation"
  Constant1/1 -> Bus Creator/2  "Height Breakpoints"
  Constant2/1 -> Bus Creator/3  "Pressure Breakpoints"
  Constant3/1 -> Bus Creator/4  "Temperature Breakpoints"
  Constant4/1 -> Bus Creator/5  "Wind Direction Breakpoints"
  Constant5/1 -> Bus Creator/6  "Wind Speed Breakpoints"

== system AirbrakeFlightSim/Simulate True Dynamics 6DOF/Define Vehicle ==
  note: Motor Properties
  note: Fins
  note: Geometric Properties
  note: Mass Properties
  note: Vehicle Mass in unloaded
      | configuration
  Bus Creator : BusCreator  Inputs=Vehicle Mass [kg],Vehicle Inertia [kg-m2],CG2CP Vector [m],Cross Sectional Area [m2],Number of Fins,Fin C_N_alpha,Fin Planform Area [m2],Motor Thrust Breakpoints,Motor Mass Breakpoints,Motor Time Breakpoints
  CG2CP Vector [m] : Constant  Value=[-0.5 0 0]
  Cross Sectional Area [m2] : Constant  Value=0.0154675624916256
  Fin C_N_alpha : Constant  Value=2.316
  Fin Planform Area [m2] : Constant  Value=0.02049724
  Motor Mass Breakpoints : Constant  Value=|
      | [   3.8555e+00
      |    3.8464e+00
      |    3.8325e+00
      |    3.8156e+00
      |    3.7411e+00
      |    3.5246e+00
      |    3.2573e+00
      |    2.9946e+00
      |    2.6223e+00
      |    2.3868e+00
      |    2.1980e+00
      |    2.1014e+00
      |    2.0699e+00
      |    2.0616e+00
      |    2.0533e+00
      |    2.0440e+00
      |    2.0356e+00
      |    2.0334e+00
      |    2.0321e+00
      |    2.0321e+00]
  Motor Thrust Breakpoints : Constant  Value=|
      | [   4.8137e+01
      |    2.1073e+03
      |    2.2892e+03
      |    2.1501e+03
      |    2.1020e+03
      |    2.1501e+03
      |    2.1555e+03
      |    2.1180e+03
      |    2.0004e+03
      |    1.8987e+03
      |    1.8399e+03
      |    1.8185e+03
      |    1.6527e+03
      |    1.3746e+03
      |    9.3600e+02
      |    5.3486e+02
      |    2.4069e+02
      |    1.1232e+02
      |    5.3490e+00
      |             0]
  Motor Time Breakpoints : Constant  Value=|
      | [   2.0000e-02
      |    4.0000e-02
      |    5.5000e-02
      |    7.3000e-02
      |    1.5600e-01
      |    3.9700e-01
      |    6.9100e-01
      |    9.8200e-01
      |    1.4100e+00
      |    1.6960e+00
      |    1.9350e+00
      |    2.0600e+00
      |    2.1030e+00
      |    2.1160e+00
      |    2.1330e+00
      |    2.1630e+00
      |    2.2140e+00
      |    2.2440e+00
      |    2.2960e+00
      |    2.3090e+00]
  Number of Fins : Constant  Value=3
  Vehicle Inertia [kg-m2] : Constant  Value=[9.2e-2 0 0; 0 19 0; 0 0 19]
  Vehicle Mass [kg] : Constant  Value=16.66100115
  Vehicle Properties : Outport
  wires:
  Vehicle Mass [kg]/1 -> Bus Creator/1  "Vehicle Mass [kg]"
  Vehicle Inertia [kg-m2]/1 -> Bus Creator/2  "Vehicle Inertia [kg-m2]"
  CG2CP Vector [m]/1 -> Bus Creator/3  "CG2CP Vector [m]"
  Cross Sectional Area [m2]/1 -> Bus Creator/4  "Cross Sectional Area [m2]"
  Number of Fins/1 -> Bus Creator/5  "Number of Fins"
  Fin C_N_alpha/1 -> Bus Creator/6  "Fin C_N_alpha"
  Fin Planform Area [m2]/1 -> Bus Creator/7  "Fin Planform Area [m2]"
  Motor Thrust Breakpoints/1 -> Bus Creator/8  "Motor Thrust Breakpoints"
  Motor Mass Breakpoints/1 -> Bus Creator/9  "Motor Mass Breakpoints"
  Motor Time Breakpoints/1 -> Bus Creator/10  "Motor Time Breakpoints"
  Bus Creator/1 -> Vehicle Properties/1  "Vehicle Properties"

== system AirbrakeFlightSim/Simulate True Dynamics 6DOF/Initial Conditions ==
  note: Initial State Vector
  note: Launch Rail Conditions
  Azimuth [deg] : Constant  Value=0
  Bus Creator : BusCreator  Inputs=Initial State
  Degrees to Radians : simulink_extras/Transformations/Degrees to Radians
  Degrees to Radians1 : simulink_extras/Transformations/Degrees to Radians
  Elevation [deg] : Constant  Value=85
  Mux : Mux  Inputs=12
  p0 : Constant  Value=0
  p_down_0 : Constant  Value=0
  p_east_0 : Constant  Value=0
  p_north_0 : Constant  Value=0
  phi0 : Constant  Value=0
  q0 : Constant  Value=0
  r0 : Constant  Value=0
  u0 : Constant  Value=0
  v0 : Constant  Value=0
  w0 : Constant  Value=0
  Out1 : Outport
  wires:
  u0/1 -> Mux/1
  v0/1 -> Mux/2
  w0/1 -> Mux/3
  p0/1 -> Mux/4
  q0/1 -> Mux/5
  r0/1 -> Mux/6
  Azimuth [deg]/1 -> Degrees to Radians/1
  p_north_0/1 -> Mux/10
  p_east_0/1 -> Mux/11
  p_down_0/1 -> Mux/12
  Elevation [deg]/1 -> Degrees to Radians1/1
  phi0/1 -> Mux/7
  Bus Creator/1 -> Out1/1
  Mux/1 -> Bus Creator/1  "Initial State"
  Degrees to Radians/1 -> Mux/9  "psi0"
  Degrees to Radians1/1 -> Mux/8  "theta0"

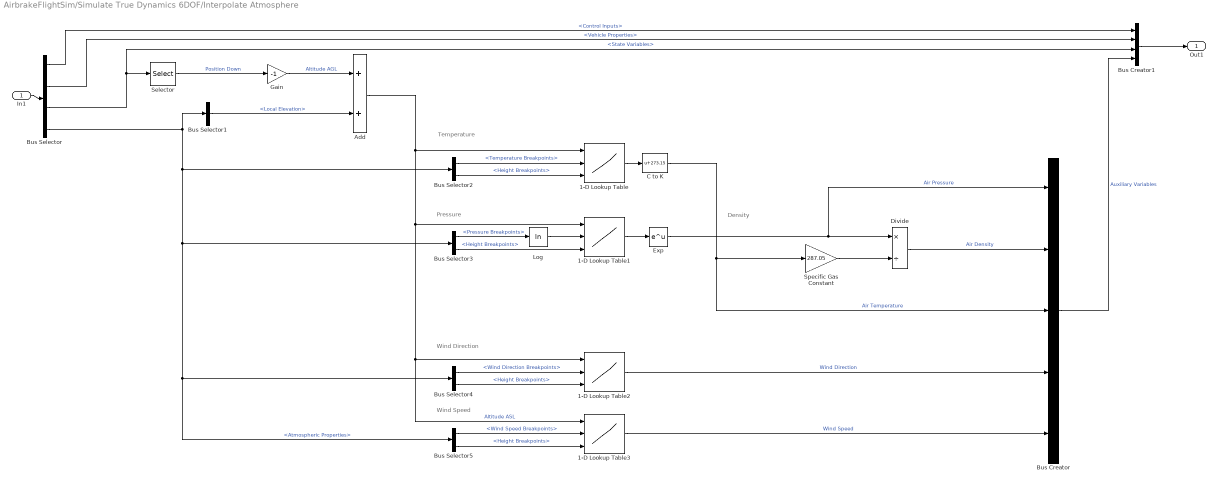
== system AirbrakeFlightSim/Simulate True Dynamics 6DOF/Interpolate Atmosphere ==
  note: Wind Direction
  note: Density
  note: Temperature
  note: Pressure
  note: Wind Speed
  In1 : Inport
  1-D Lookup Table{,1..3} (4 alike) : Lookup_n-D  NumberOfTableDimensions=1  BreakpointsForDimension1Source=Input port  BreakpointsForDimension1=[-5:5]  TableSource=Input port  Table=tanh([-5:5])  InternalRulePriority=Speed  RndMeth=Simplest
      settings: InputPortMap=u0,p221,p5
  Add : Sum
  Bus Creator : BusCreator  Inputs=5
  Bus Creator1 : BusCreator  Inputs=Control Inputs,Vehicle Properties,State Variables,Auxiliary Variables
  Bus Selector : BusSelector  OutputSignals=Control Inputs,Vehicle Properties,State Variables,Atmospheric Properties
  Bus Selector1 : BusSelector  OutputSignals=Local Elevation
  Bus Selector2 : BusSelector  OutputSignals=Temperature Breakpoints,Height Breakpoints
  Bus Selector3 : BusSelector  OutputSignals=Pressure Breakpoints,Height Breakpoints
  Bus Selector4 : BusSelector  OutputSignals=Wind Direction Breakpoints,Height Breakpoints
  Bus Selector5 : BusSelector  OutputSignals=Wind Speed Breakpoints,Height Breakpoints
  C to K : Bias  Bias=273.15  SaturateOnIntegerOverflow=off
  Divide : Product  Inputs=*/
  Exp : Math
  Gain : Gain  Gain=-1
  Log : Math  Operator=log
  Selector : Selector  InputPortWidth=12  IndexOptions=Index vector (dialog)  Indices=[12]  OutputSizes=1
  Specific Gas Constant : Gain  Gain=287.05
  Out1 : Outport
  wires:
  In1/1 -> Bus Selector/1
  Bus Selector/3 -> Bus Creator1/3, Selector/1  "<State Variables>"
  Selector/1 -> Gain/1  "Position Down"
  Gain/1 -> Add/1  "Altitude AGL"
  Bus Selector/4 -> Bus Selector1/1, Bus Selector2/1, Bus Selector5/1, Bus Selector4/1, Bus Selector3/1  "<Atmospheric Properties>"
  Bus Selector1/1 -> Add/2  "<Local Elevation>"
  Add/1 -> 1-D Lookup Table1/1, 1-D Lookup Table3/1, 1-D Lookup Table2/1, 1-D Lookup Table/1  "Altitude ASL"
  Bus Selector2/1 -> 1-D Lookup Table/2  "<Temperature Breakpoints>"
  Bus Selector2/2 -> 1-D Lookup Table/3  "<Height Breakpoints>"
  Bus Selector3/2 -> 1-D Lookup Table1/3  "<Height Breakpoints>"
  1-D Lookup Table1/1 -> Exp/1
  Specific Gas Constant/1 -> Divide/2
  1-D Lookup Table/1 -> C to K/1
  Exp/1 -> Bus Creator/1, Divide/1  "Air Pressure"
  Bus Creator1/1 -> Out1/1
  Bus Selector/2 -> Bus Creator1/2  "<Vehicle Properties>"
  Bus Selector/1 -> Bus Creator1/1  "<Control Inputs>"
  Bus Creator/1 -> Bus Creator1/4  "Auxiliary Variables"
  Bus Selector3/1 -> Log/1  "<Pressure Breakpoints>"
  Log/1 -> 1-D Lookup Table1/2
  C to K/1 -> Bus Creator/3, Specific Gas Constant/1  "Air Temperature"
  Divide/1 -> Bus Creator/2  "Air Density"
  Bus Selector4/1 -> 1-D Lookup Table2/2  "<Wind Direction Breakpoints>"
  Bus Selector4/2 -> 1-D Lookup Table2/3  "<Height Breakpoints>"
  Bus Selector5/1 -> 1-D Lookup Table3/2  "<Wind Speed Breakpoints>"
  Bus Selector5/2 -> 1-D Lookup Table3/3  "<Height Breakpoints>"
  1-D Lookup Table2/1 -> Bus Creator/4  "Wind Direction"
  1-D Lookup Table3/1 -> Bus Creator/5  "Wind Speed"

== system AirbrakeFlightSim/Simulate True Dynamics 6DOF/Interpolate Thrust & Mass ==
  In1 : Inport
  Bus Creator : BusCreator  Inputs=Simulation Time,Vehicle Properties,Atmospheric Properties
  Bus Creator1 : BusCreator  Inputs=Simulation Time,Thrust,Mass,Inertia
  Bus Selector : BusSelector  OutputSignals=Simulation Time
  Bus Selector1 : BusSelector  OutputSignals=Vehicle Properties,Atmospheric Properties
  Check Motor Burnout : Subsystem
  Clock : Clock
  Inertia (UNFINISHED) : Subsystem
  Interpolate Mass : Subsystem
  Interpolate Thrust : Subsystem
  Out1 : Outport
  wires:
  Bus Creator/1 -> Check Motor Burnout/1(In1), Inertia (UNFINISHED)/1(In1), Interpolate Mass/1(1), Bus Selector/1, Interpolate Thrust/1(In1)
  Bus Creator1/1 -> Out1/1
  In1/1 -> Bus Selector1/1
  Bus Selector1/1 -> Bus Creator/2  "<Vehicle Properties>"
  Bus Selector1/2 -> Bus Creator/3  "<Atmospheric Properties>"
  Clock/1 -> Bus Creator/1  "Simulation Time"
  Interpolate Mass/1(Mass) -> Bus Creator1/3  "Mass"
  Interpolate Thrust/1(Out1) -> Bus Creator1/2  "Thrust"
  Inertia (UNFINISHED)/1(Out1) -> Bus Creator1/4  "Inertia"
  Bus Selector/1 -> Bus Creator1/1  "<Simulation Time>"

== system AirbrakeFlightSim/Simulate True Dynamics 6DOF/Net Force ==
  In1 : Inport
  In2 : Inport  Port=2
  Add : Sum
  Bus Creator : BusCreator  Inputs=Aerodynamic Forces (Wind Axes),Angle of Attack,Angle of Sideslip,Dynamic Pressure,Mach Number,Speed of Sound,Air Pressure,Air Density,Air Temperature,Net Force,Simulation Time,Thrust,Mass,Inertia
  Bus Creator1 : BusCreator  Inputs=Vehicle Properties,Auxiliary Variables
  Bus Selector : BusSelector  OutputSignals=Auxiliary Variables.Angle of Attack,Auxiliary Variables.Angle of Sideslip,Auxiliary Variables.Aerodynamic Forces (Wind Axes)
  Bus Selector1 : BusSelector  OutputSignals=Thrust
  Bus Selector2 : BusSelector  OutputSignals=Auxiliary Variables.Aerodynamic Forces (Wind Axes),Auxiliary Variables.Angle of Attack,Auxiliary Variables.Angle of Sideslip,Auxiliary Variables.Dynamic Pressure,Auxiliary Variables.Mach Number,Auxiliary Variables.Speed of Sound,Auxiliary Variables.Air Pressure,Auxiliary Variables.Air Density,Auxiliary Variables.Air Temperature
  Bus Selector3 : BusSelector  OutputSignals=Vehicle Properties
  Bus Selector4 : BusSelector  OutputSignals=Simulation Time,Thrust,Mass,Inertia
  Gain : Gain  Gain=[1 0 0]'
  MATLAB Function : MATLAB Function  TreatAsAtomicUnit=on
  Out1 : Outport
  wires:
  In1/1 -> Bus Selector2/1, Bus Selector3/1, Bus Selector/1
  Bus Selector/3 -> MATLAB Function/3(aero_w_N)  "<Aerodynamic Forces (Wind Axes)>"
  Bus Selector/2 -> MATLAB Function/2(beta_rad)  "<Angle of Sideslip>"
  Bus Selector/1 -> MATLAB Function/1(alpha_rad)  "<Angle of Attack>"
  In2/1 -> Bus Selector4/1, Bus Selector1/1
  Bus Selector1/1 -> Gain/1  "<Thrust>"
  Gain/1 -> Add/2
  MATLAB Function/1(aero_b_N) -> Add/1
  Bus Selector2/1 -> Bus Creator/1  "<Aerodynamic Forces (Wind Axes)>"
  Bus Selector2/2 -> Bus Creator/2  "<Angle of Attack>"
  Bus Selector2/3 -> Bus Creator/3  "<Angle of Sideslip>"
  Bus Selector2/4 -> Bus Creator/4  "<Dynamic Pressure>"
  Bus Selector2/5 -> Bus Creator/5  "<Mach Number>"
  Bus Selector2/6 -> Bus Creator/6  "<Speed of Sound>"
  Bus Selector2/7 -> Bus Creator/7  "<Air Pressure>"
  Bus Selector2/8 -> Bus Creator/8  "<Air Density>"
  Bus Selector2/9 -> Bus Creator/9  "<Air Temperature>"
  Bus Selector3/1 -> Bus Creator1/1  "<Vehicle Properties>"
  Bus Creator/1 -> Bus Creator1/2  "Auxiliary Variables"
  Bus Creator1/1 -> Out1/1
  Add/1 -> Bus Creator/10  "Net Force"
  Bus Selector4/1 -> Bus Creator/11  "<Simulation Time>"
  Bus Selector4/2 -> Bus Creator/12  "<Thrust>"
  Bus Selector4/3 -> Bus Creator/13  "<Mass>"
  Bus Selector4/4 -> Bus Creator/14  "<Inertia>"

== system AirbrakeFlightSim/Simulate True Dynamics 6DOF/Net Moment ==
  In1 : Inport
  Bus Creator : BusCreator  Inputs=Net Moment,Aerodynamic Forces (Wind Axes),Angle of Attack,Angle of Sideslip,Dynamic Pressure,Mach Number,Speed of Sound,Air Pressure,Air Density,Air Temperature,Net Force,Simulation Time,Thrust,Mass,Inertia
  Bus Selector : BusSelector  OutputSignals=Vehicle Properties.CG2CP Vector [m],Auxiliary Variables.Net Force
  Bus Selector1 : BusSelector  OutputSignals=Auxiliary Variables.Aerodynamic Forces (Wind Axes),Auxiliary Variables.Angle of Attack,Auxiliary Variables.Angle of Sideslip,Auxiliary Variables.Dynamic Pressure,Auxiliary Variables.Mach Number,Auxiliary Variables.Speed of Sound,Auxiliary Variables.Air Pressure,Auxiliary Variables.Air Density,Auxiliary Variables.Air Temperature,Auxiliary Variables.Net Force,Auxiliary Variables.Simulation Time,Auxiliary Variables.Thrust,Auxiliary Variables.Mass,Auxiliary Variables.Inertia
  Cross Product : matrix_library/Cross Product
  Out1 : Outport
  wires:
  In1/1 -> Bus Selector1/1, Bus Selector/1
  Bus Selector/1 -> Cross Product/1  "<CG2CP Vector [m]>"
  Bus Selector/2 -> Cross Product/2  "<Net Force>"
  Bus Selector1/1 -> Bus Creator/2  "<Aerodynamic Forces (Wind Axes)>"
  Bus Selector1/2 -> Bus Creator/3  "<Angle of Attack>"
  Bus Selector1/3 -> Bus Creator/4  "<Angle of Sideslip>"
  Bus Selector1/4 -> Bus Creator/5  "<Dynamic Pressure>"
  Bus Selector1/5 -> Bus Creator/6  "<Mach Number>"
  Bus Selector1/6 -> Bus Creator/7  "<Speed of Sound>"
  Bus Selector1/7 -> Bus Creator/8  "<Air Pressure>"
  Bus Selector1/8 -> Bus Creator/9  "<Air Density>"
  Bus Selector1/9 -> Bus Creator/10  "<Air Temperature>"
  Bus Selector1/10 -> Bus Creator/11  "<Net Force>"
  Bus Selector1/11 -> Bus Creator/12  "<Simulation Time>"
  Bus Selector1/12 -> Bus Creator/13  "<Thrust>"
  Bus Selector1/13 -> Bus Creator/14  "<Mass>"
  Cross Product/1 -> Bus Creator/1  "Net Moment"
  Bus Creator/1 -> Out1/1
  Bus Selector1/14 -> Bus Creator/15  "<Inertia>"

== system AirbrakeFlightSim/Simulate True Dynamics 6DOF/Stop Integration ==
  note: Apogee Event
  note: Landing Event
  In1 : Inport
  Add Constant : Bias  Bias=+0.1  SaturateOnIntegerOverflow=off
  Add Constant1 : Bias  Bias=+1  SaturateOnIntegerOverflow=off
  Bus Selector : BusSelector  OutputSignals=State Variables,State Derivatives
  Constant : Constant  Value=0
  Constant1 : Constant  Value=0
  Gain : Gain  Gain=-1
  Gain1 : Gain  Gain=-1
  Manual Switch : ManualSwitch
  Relational Operator : RelationalOperator  Operator=<=  OutDataTypeStr=boolean  RndMeth=Simplest  InputSameDT=off
  Relational Operator1 : RelationalOperator  Operator=<=  OutDataTypeStr=boolean  RndMeth=Simplest  InputSameDT=off
  Selector : Selector  InputPortWidth=12  IndexOptions=Index vector (dialog)  Indices=[12]  OutputSizes=1
  Selector1 : Selector  InputPortWidth=12  IndexOptions=Index vector (dialog)  Indices=[12]  OutputSizes=1  RuntimeRangeChecks=on
  Stop Simulation : Stop
  wires:
  Selector/1 -> Gain/1
  Gain/1 -> Add Constant/1
  Add Constant/1 -> Relational Operator/1
  Constant/1 -> Relational Operator/2
  Selector1/1 -> Gain1/1
  Add Constant1/1 -> Relational Operator1/1
  Constant1/1 -> Relational Operator1/2
  Relational Operator/1 -> Manual Switch/1
  Relational Operator1/1 -> Manual Switch/2
  Manual Switch/1 -> Stop Simulation/1
  In1/1 -> Bus Selector/1
  Bus Selector/1 -> Selector/1  "<State Variables>"
  Bus Selector/2 -> Selector1/1  "<State Derivatives>"
  Gain1/1 -> Add Constant1/1

== system AirbrakeFlightSim/Navigation/Compute Drag/Reorganize ==
  nav : Inport
  y : Inport  Port=2
  Bus Creator : BusCreator  Inputs=3
  Bus Selector : BusSelector  OutputSignals=NED,Estimated State
  dragConstant : Outport
  wires:
  nav/1 -> Bus Selector/1
  Bus Selector/1 -> Bus Creator/1  "<NED>"
  Bus Selector/2 -> Bus Creator/2  "<Estimated State>"
  y/1 -> Bus Creator/3  "Estimated Drag Constant"
  Bus Creator/1 -> dragConstant/1

== system AirbrakeFlightSim/Simulate Sensors/Ideal Sensors/Altimeter ==
  x,xdot : Inport
  Bus Selector : BusSelector  OutputSignals=State Variables
  Gain : Gain  Gain=-1
  Selector : Selector  InputPortWidth=12  IndexOptions=Index vector (dialog)  Indices=[12]  OutputSizes=1
  altitudehat : Outport
  wires:
  Selector/1 -> Gain/1  "p_down_m"
  Gain/1 -> altitudehat/1  "altitude"
  x,xdot/1 -> Bus Selector/1
  Bus Selector/1 -> Selector/1  "<State Variables>"

== system AirbrakeFlightSim/Simulate Sensors/Ideal Sensors/GPS ==
  x,xdot : Inport
  Bus Selector : BusSelector  OutputSignals=State Variables,State Derivatives
  Selector : Selector  InputPortWidth=12  IndexOptions=Index vector (dialog)  Indices=[10 11 12]  OutputSizes=1
  Selector1 : Selector  InputPortWidth=12  IndexOptions=Index vector (dialog)  Indices=[10 11 12]  OutputSizes=1
  rhat : Outport
  vhat : Outport  Port=2
  wires:
  x,xdot/1 -> Bus Selector/1
  Bus Selector/1 -> Selector/1  "<State Variables>"
  Bus Selector/2 -> Selector1/1  "<State Derivatives>"
  Selector1/1 -> vhat/1  "Measured GPS Velocity"
  Selector/1 -> rhat/1  "Measured GPS Position"
